simulink model "traffic_intersection_arduino"  (R2025b)
settings: Solver=FixedStepAuto  StartTime=0.0  StopTime=Inf  RelTol=1e-3  EnableMultiTasking=on
libraries: arduinolib x8, simulink x1, arduinosensorlib x1
settings Model: ExtModeTrigDuration=2  Creator=kathyz  LastModifiedBy=kathyz
settings SolverCC: AutoInsertRateTranBlk=on
settings OptimizationCC: EnhancedBackFolding=on  PassReuseOutputArgsAs=Individual arguments  ZeroExternalMemoryAtStartup=off  ZeroInternalMemoryAtStartup=off  MaxStackSize=64  OptimizeBlockOrder=speed  DifferentSizesBufferReuse=on  OptimizationCustomize=off  EfficientTunableParamExpr=on
settings DebuggingCC: ParameterTunabilityLossMsg=error
settings HardwareCC: ProdBitPerInt=16.0  ProdBitPerPointer=16.0  ProdBitPerSizeT=16.0  ProdBitPerPtrDiffT=16.0  ProdLargestAtomicFloat=None  ProdWordSize=8.0  ProdHWDeviceType=Atmel->AVR
settings SFSimCC: MATLABDynamicMemAlloc=off
settings RTWCC: SystemTargetFile=ert.tlc  HardwareBoard=Arduino Mega 2560  TemplateMakefile=ert_default_tmf  Toolchain=Arduino AVR  BuildConfiguration=Faster Runs  Description=Embedded Coder
settings CodeAppCC: ForceParamTrailComments=on  IgnoreCustomStorageClasses=off  OperatorAnnotations=on  SimulinkDataObjDesc=on  SFDataObjDesc=on  InsertBlockDesc=on
settings ERTTargetCC: ExtModeTransport=3.0  ExtModeStaticAlloc=on  ExtModeAutomaticAllocSize=off  ExtModeStaticAllocSize=2048.0  ExtModeMexFile=ext_xcp  ExtModeIntrfLevel=Level2 - Open  InlinedParameterPlacement=Hierarchical  SupportContinuousTime=on  SupportVariableSizeSignals=on

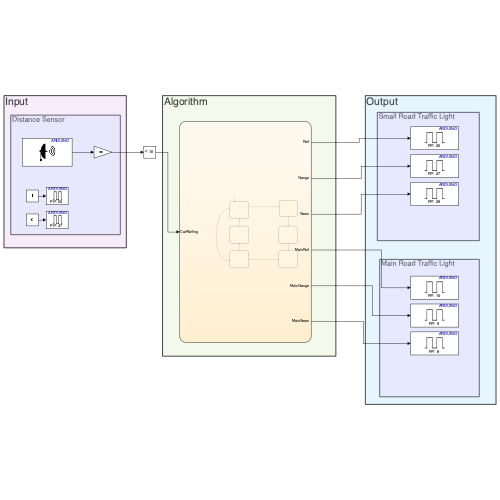
[thumbnail: Simulink's stored preview of the top-level diagram]
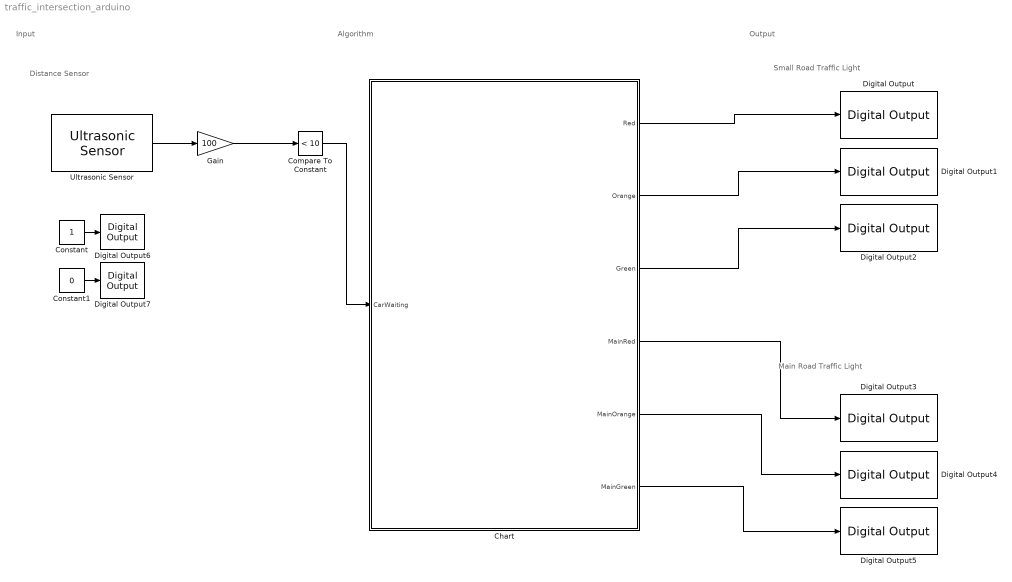
== system traffic_intersection_arduino ==
  note: Algorithm
  note: Output
  note: Small Road Traffic Light
  note: Main Road Traffic Light
  note: Input
  note: Distance Sensor
  Chart : Stateflow chart  TreatAsAtomicUnit=on
  Compare To Constant : simulink/Logic and Bit Operations/Compare To Constant  relop=<  const=10  OutDataTypeStr=boolean
  Constant : Constant
  Constant1 : Constant  Value=0
  Digital Output : arduinolib/Digital Output  pinNumber=25  Direction=output  blockPlatform=arduino
  Digital Output1 : arduinolib/Digital Output  pinNumber=27  Direction=output  blockPlatform=arduino
  Digital Output2 : arduinolib/Digital Output  pinNumber=29  Direction=output  blockPlatform=arduino
  Digital Output3 : arduinolib/Digital Output  pinNumber=10  Direction=output  blockPlatform=arduino
  Digital Output4 : arduinolib/Digital Output  pinNumber=9  Direction=output  blockPlatform=arduino
  Digital Output5 : arduinolib/Digital Output  pinNumber=8  Direction=output  blockPlatform=arduino
  Digital Output6 : arduinolib/Digital Output  pinNumber=53  Direction=output  blockPlatform=arduino
  Digital Output7 : arduinolib/Digital Output  pinNumber=47  Direction=output  blockPlatform=arduino
  Gain : Gain  Gain=100
  Ultrasonic Sensor : arduinosensorlib/Ultrasonic Sensor  NumSignalPins=2  TrigPin=51  EchoPin=49  SignalPin=3  SampleTime_=0.1  blockPlatform=ARDUINO
  wires:
  Ultrasonic Sensor/1 -> Gain/1
  Gain/1 -> Compare To Constant/1
  Constant1/1 -> Digital Output7/1
  Constant/1 -> Digital Output6/1
  Chart/1(Red) -> Digital Output/1
  Chart/2(Orange) -> Digital Output1/1
  Chart/3(Green) -> Digital Output2/1
  Chart/4(MainRed) -> Digital Output3/1
  Chart/5(MainOrange) -> Digital Output4/1
  Chart/6(MainGreen) -> Digital Output5/1
  Compare To Constant/1 -> Chart/1(CarWaiting)

== stateflow chart traffic_intersection_arduino/Chart ==
  state Green
    Red=0;
    Orange=0;
    Green=1;
    MainRed=1;
    MainOrange=0;
    MainGreen=0;
  state MainRed
    Red=1;
    Orange=0;
    Green=0;
    MainRed=1;
    MainOrange=0;
    MainGreen=0;
  state MainOrange
    Red=1;
    Orange=0;
    Green=0;
    MainRed=0;
    MainOrange=1;
    MainGreen=0;
  state Orange
    Red=0;
    Orange=1;
    Green=0;
    MainRed=1;
    MainOrange=0;
    MainGreen=0;
  state MainGreen
    Red=1;
    Orange=0;
    Green=0;
    MainRed=0;
    MainOrange=0;
    MainGreen=1;
  state Red
    Red=1;
    Orange=0;
    Green=0;
    MainRed=1;
    MainOrange=0;
    MainGreen=0;
  (default) -> MainRed
  MainRed -> Green [order 1] : [after(1,sec)&CarWaiting]
  MainRed -> MainGreen [order 2] : [after(2,sec)&~CarWaiting]
  Green -> Orange : after(3,sec)
  MainOrange -> MainRed : after(1, sec)
  MainGreen -> MainOrange : after(3,sec)
  Orange -> Red : after(1,sec)
  Red -> MainGreen : after(2,sec)
  data: Red output; Orange output; Green output; MainRed output; MainOrange output; MainGreen output; CarWaiting input
